simulink model "UnaryMinus1"  (R2017b)
settings: Solver=FixedStepDiscrete  StartTime=0.0  StopTime=10.0  FixedStep=0.200000  RelTol=1e-3  EnableMultiTasking=on
model workspace (MAT data in the model file):
  already_pp = 0
  input_struct.time = [0; 0.2; 0.4; 0.6; 0.8; 1; 1.2; 1.4; 1.6; 1.8; 2; 2.2; 2.4; 2.6; 2.8; 3; 3.2; 3.4; 3.6; 3.8; 4; 4.2; 4.4; 4.6; 4.8; 5; 5.2; 5.4; 5.6; 5.8; 6; 6.2; 6.4; 6.6; 6.8; 7; 7.2; 7.4; 7.6; 7.8; 8; 8.2; 8.4; 8.6; 8.8; 9; 9.2; 9.4; 9.6; 9.8; 10; 10.2; 10.4; 10.6; 10.8; 11; 11.2; 11.4; 11.6; 11.8; 12; 12.2; 12.4; 12.6; 12.8; 13; 13.2; 13.4; 13.6; 13.8; 14; 14.2; 14.4; 14.6; 14.8; 15; 15.2; 15.4; 15.6; 15.8; 16; 16.2; 16.4; 16.6; 16.8; 17; 17.2; 17.4; 17.6; 17.8; 18; 18.2; 18.4; 18.6; 18.8; 19; 19.2; 19.4; 19.6; 19.8]
  input_struct.signals(1).name = 'In1'
  input_struct.signals(1).values = [20; -96; 80; -9; -89; -79; 100; 74; 23; -95; -36; -7; -81; 14; -35; -10; 16; -85; -89; -40; 4; 12; -52; 83; 65; -11; 97; 16; -53; 62; -10; -50; 92; -72; 3; 95; 30; 23; -6; 16; 83; -25; -55; -15; -46; -11; 26; 7; -23; 75; -40; -20; 4; -88; -54; -77; -81; 78; -94; 68; 1; -78; -2; 20; -82; 96; 31; -8; 73; -48; 65; -34; 89; -51; 92; 2; 13; 99; 54; -37; -89; -92; 63; -18; -23; 5; 79; -19; 21; -81; -33; -71; -51; -24; -46; -57; 27; 60; -59; 80]
  input_struct.signals(1).dimensions = 1
  input_struct.signals(2).name = 'In2'
  input_struct.signals(2).values = [49.1418941611; 7.2771614077; 93.9930388039; 12.9766340355; -56.4620202112; 71.5526573691; 72.3998635655; -37.3395610327; -34.6031577005; 68.0026808037; -1.49344274697; -89.6195031824; 55.6036737893; -14.6655228354; -44.0076237227; -33.2983976374; -26.6120095907; 58.9584820424; -92.2618428865; 45.3338670991; 74.5368918601; -42.8370434935; 31.3698518771; -53.6226749801; 24.3907883089; -84.9752465293; 93.3511750999; 21.9939913248; -23.2569640491; -93.8860453317; 71.513117363; 20.7086370763; 69.5680810182; 0.923249375269; -98.4178324853; 83.8146354929; -17.8590408694; 46.4731495571; -69.7789442279; 63.0466553374; 81.9205063722; 55.5884922366; 51.4246272851; -18.9604952918; 40.3802160342; 13.0921874243; 16.9472703847; -31.0170801465; 40.8466479001; -67.8272641955; -99.6972133266; 12.4001704282; 9.2968249888; 10.1655523643; 38.9073521589; 85.4988184109; 88.8420617736; 80.6526658651; 20.8212572783; 85.2419513967; -76.6107483176; -31.8396984209; -92.6539112833; 7.67397009844; 47.445760245; -63.7554994691; -14.7506676887; -80.3664085942; -39.3556866642; 56.024522393; 7.39208334386; 53.8142865949; 27.7887291257; 78.6296491316; -87.8619225133; -64.8456908463; -16.7336281957; 47.9583681963; 78.5909584981; -94.8293386822; -72.4873943247; -15.1825134742; 52.9133563758; 4.88743753036; 50.8962717899; -66.0403113243; 34.5454011823; 23.7305485492; -98.6307821078; 48.0451048275; 98.3470955904; -74.3637285525; -27.8834479449; -61.7853469255; 42.8795321628; -64.4265977463; 97.3697499971; -96.6001740197; -92.0407060861; 60.866106387]
  input_struct.signals(2).dimensions = 1
settings Model: Creator=Teme  LastModifiedBy=hbourbou
settings DataIOCC: LimitDataPoints=on  SaveFormat=Structure
settings OptimizationCC: LifeSpan=inf
settings DebuggingCC: AlgebraicLoopMsg=error  ArtificialAlgebraicLoopMsg=error  SFUnexpectedBacktrackingDiag=warning  SFNoUnconditionalDefaultTransitionDiag=warning  SFExecutionAtInitializationDiag=none
settings HardwareCC: ProdBitPerPointer=32  ProdBitPerSizeT=32  ProdBitPerPtrDiffT=32  ProdLargestAtomicFloat=None  ProdIntDivRoundTo=Undefined  ProdEndianess=Unspecified  ProdWordSize=32  ProdHWDeviceType=32-bit Generic
settings ModelReferenceCC: PropagateSignalLabelsOutOfModel=off
settings RTWCC: Toolchain=Clang v3.1 | gmake (64-bit Mac)
settings CodeAppCC: StateflowObjectComments=on
settings GRTTargetCC: TargetLangStandard=C89/C90 (ANSI)  GeneratePreprocessorConditionals=Disable all
settings ConfigComp: CovMetricSettings=dw  CovHtmlReporting=on  CovSaveCumulativeToWorkspaceVar=on  CovSaveSingleToWorkspaceVar=on  CovExternalEMLEnable=off

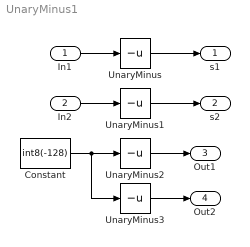
== system UnaryMinus1 ==
  In1 : Inport  OutDataTypeStr=int8  PortDimensions=1
  In2 : Inport  Port=2  OutDataTypeStr=double  PortDimensions=1
  Constant : Constant  Value=int8(-128)
  UnaryMinus : UnaryMinus  SaturateOnIntegerOverflow=on
  UnaryMinus1 : UnaryMinus
  UnaryMinus2 : UnaryMinus  SaturateOnIntegerOverflow=on
  UnaryMinus3 : UnaryMinus
  s1 : Outport
  s2 : Outport  Port=2
  Out1 : Outport  Port=3
  Out2 : Outport  Port=4
  wires:
  UnaryMinus/1 -> s1/1
  In1/1 -> UnaryMinus/1
  In2/1 -> UnaryMinus1/1
  UnaryMinus1/1 -> s2/1
  Constant/1 -> UnaryMinus3/1, UnaryMinus2/1
  UnaryMinus2/1 -> Out1/1
  UnaryMinus3/1 -> Out2/1
